simulink model "P5_5_InvertedPendulum"  (R2025b)
settings: Solver=VariableStepAuto  StartTime=0.0  StopTime=10.0  MaxStep=1e-2  RelTol=1e-3
settings Model: Creator=tongx  LastModifiedBy=tongx

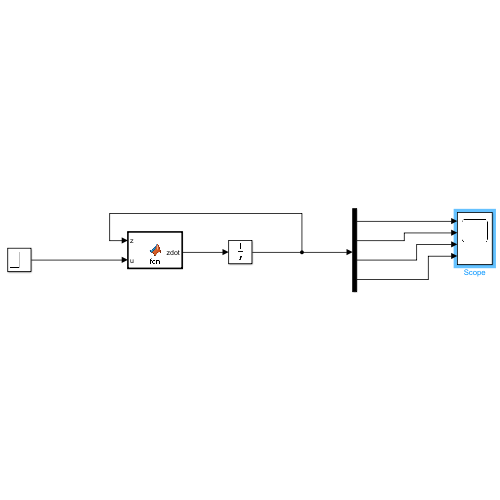
[thumbnail: Simulink's stored preview of the top-level diagram]
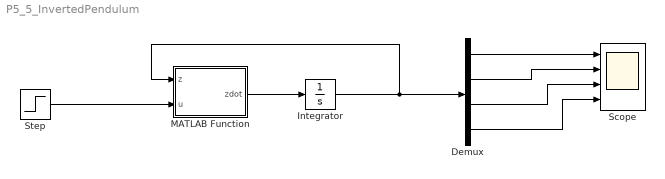
== system P5_5_InvertedPendulum ==
  Demux : Demux
  Integrator : Integrator  InitialCondition=[0 0 0 0].';
  MATLAB Function : MATLAB Function  TreatAsAtomicUnit=on
  Scope : Scope  NumInputPorts=4
      settings: ActiveDisplayYMinimum=-5.0449454777348768  ActiveDisplayYMaximum=45.4045092996139
  Step : Step  SampleTime=0
  wires:
  MATLAB Function/1(zdot) -> Integrator/1
  Integrator/1 -> Demux/1, MATLAB Function/1(z)
  Step/1 -> MATLAB Function/2(u)
  Demux/2 -> Scope/2
  Demux/1 -> Scope/1
  Demux/3 -> Scope/3
  Demux/4 -> Scope/4

== matlab function P5_5_InvertedPendulum/MATLAB Function ==
  data: z input; u input; zdot output
function zdot = fcn(z, u)

m = 0.5;
M = 0.5;
l = 0.3;
g = 9.81;

x = z(1);
theta = z(3);
theta_dt = z(4);

cth = cos(theta);
sth = sin(theta);



x_ddt = (u + m*l*sth*theta_dt.^2 - m*g*cth*sth)/(M + m - m*cth.^2);

theta_ddt = (u*cth - (M+m)*g*sth + m*l*sth*cth*theta_dt.^2)/(m*l*cth.^2 - (M+m)*l);

zdot = [z(2) x_ddt theta_dt theta_ddt].';
